simulink model "verticalFlightModel"  (R2025a)
settings: Solver=VariableStepAuto  StartTime=0.0  StopTime=10.0  RelTol=1e-3
settings Model: Creator=Ayush_S  LastModifiedBy=Ayush_S

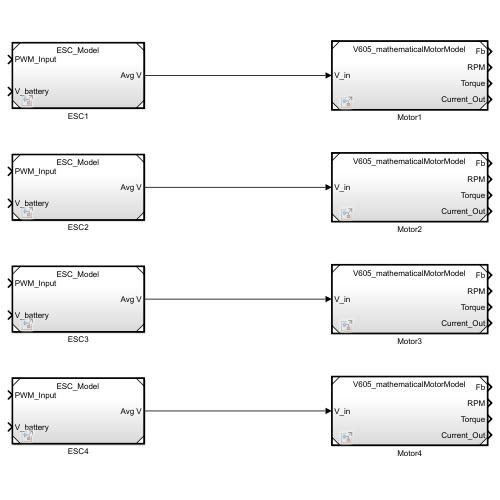
[thumbnail: Simulink's stored preview of the top-level diagram]
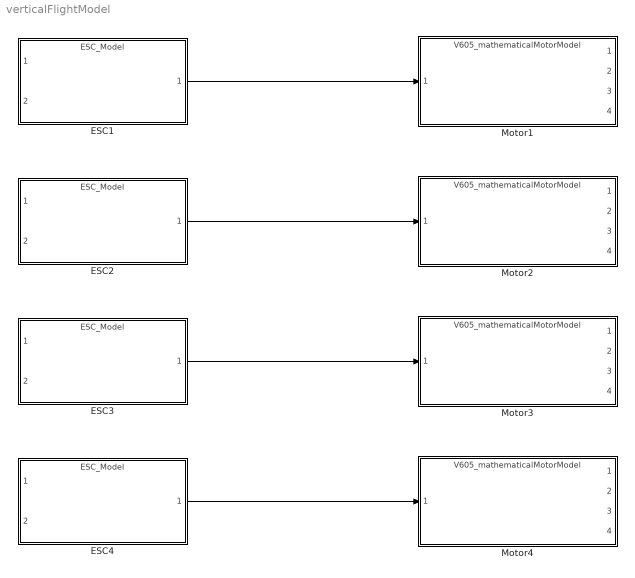
== system verticalFlightModel ==
  ESC{1..4} (4 alike) : ModelReference  ModelNameDialog=ESC_Model.slx  SimulationMode=Normal  ModelReferenceVersion=1.8
  Motor{1..4} (4 alike) : ModelReference  ModelNameDialog=V605_mathematicalMotorModel.slx  SimulationMode=Normal  ModelReferenceVersion=3.39
  wires:
  ESC1/1 -> Motor1/1
  ESC4/1 -> Motor4/1
  ESC3/1 -> Motor3/1
  ESC2/1 -> Motor2/1
